simulink model "sim_main_esb_12"  (R2018b)
settings: Solver=VariableStepAuto  StartTime=0.0  StopTime=10  RelTol=1e-3
values from neighbouring files (symbols this model uses):
  A_klm = A_sys    [main_tf_12.m]    (also in main_tf_13.m = A_sys(1:6 , 1:6))
  B_klm = B_sys    [main_tf_12.m]    (also in main_tf_13.m = B_sys(1:6 , :))
  C = 0.344    [KALMAN.m]    (also in main_sys.m = double( subs( C) ); main_sys_klm.m = double( subs( C) ); main_tf_0.m = [ 0 , 0  , Ks , ds , -Ks , -ds, 0 ]; main_tf_1.m = C_mes)
  C_klm = C_sys    [main_tf_12.m]    (also in main_tf_13.m = C_sys(: , 1:6 ))
  Ct = double( subs( Ct) )    [main_sys.m]    (also in main_sys_klm.m; main_tf_10.m; main_tf_11.m; main_tf_12.m)
  D_klm = D_sys    [main_tf_12.m]    (also in main_tf_13.m)
  sys_sys = ss(A,B,C,D)    [main_sys.m]    (also in main_sys_klm.m; main_tf_10.m; main_tf_11.m; main_tf_12.m = ss(A_sys,B_sys,C_sys_mod,D_sys_mod))
undefined symbols (not defined in the file or in its folder): Continuous, K_lq, Time
libraries: ctrlSharedLib x1
settings Model: Creator=eshojaei  LastModifiedBy=eshojaei
settings CodeAppCC: StateflowObjectComments=on

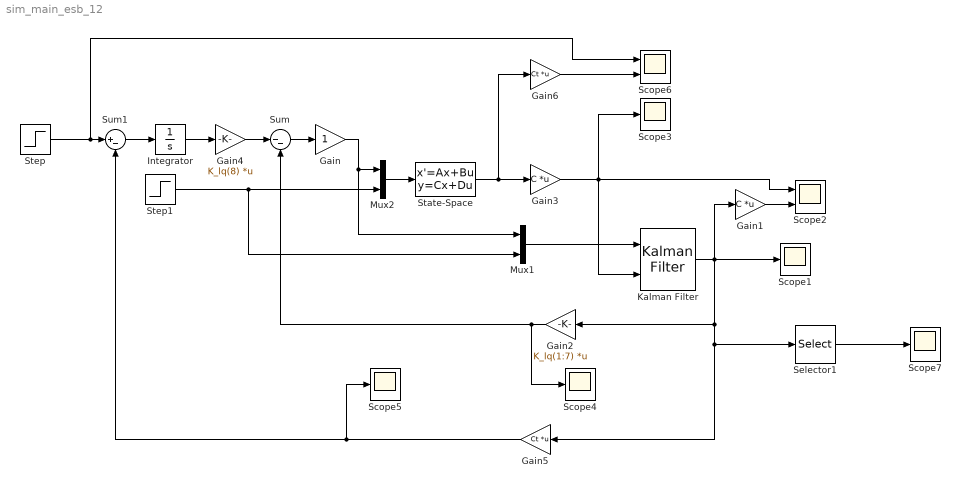
== system sim_main_esb_12 ==
  Gain : Gain
  Gain1 : Gain  Gain=C  Multiplication=Matrix(K*u)
  Gain2 : Gain  Gain=K_lq(1:7)  Multiplication=Matrix(K*u)
  Gain3 : Gain  Gain=C  Multiplication=Matrix(K*u)
  Gain4 : Gain  Gain=K_lq(8)  Multiplication=Matrix(K*u)
  Gain5 : Gain  Gain=Ct  Multiplication=Matrix(K*u)
  Gain6 : Gain  Gain=Ct  Multiplication=Matrix(K*u)
  Integrator : Integrator
  Kalman Filter : ctrlSharedLib/Kalman Filter  TimeDomain=Continuous-Time  UseCurrentEstimator=on  ModelSource=Individual A, B, C, D matrices  ModelSourceVariable=ss(0.95,1,1,0,1)  A=A_klm  B=B_klm  C=C_klm  D=D_klm  NumberOfStates=1  NumberOfInputs=1  NumberOfOutputs=1  InitialEstimateSource=Dialog  X0=0  P0=10  UseK=off  UseGH=off  NumberOfProcessNoiseInputs=1  G=1  TimeInvariantG=on  H=0  TimeInvariantH=on  Q=1  TimeInvariantQ=on  R=1  TimeInvariantR=on  N=0  TimeInvariantN=on  AddInputPort=on  AddEnablePort=off  OutputEstimatedY=off  OutputP=off  Ts=-1
      settings: SourceProductBaseCode=CT
  Mux1 : Mux  Inputs=2
  Mux2 : Mux  Inputs=2
  Scope{1,3..5,7} (5 alike) : Scope
  Scope2 : Scope  NumInputPorts=2
  Scope6 : Scope  NumInputPorts=2
  Selector1 : Selector  InputPortWidth=7  IndexOptions=Index vector (dialog)  Indices=[7]  OutputSizes=1
  State-Space : StateSpace  A=sys_sys.A  B=sys_sys.B  C=sys_sys.C  D=sys_sys.D  InitialCondition=0
  Step : Step  Time=.1  After=10  SampleTime=0
  Step1 : Step  Time=.1  After=.1  SampleTime=0
  Sum : Sum  Inputs=|--
  Sum1 : Sum  Inputs=|+-
  wires:
  Step1/1 -> Mux2/2, Mux1/2
  Gain3/1 -> Scope3/1, Scope2/1, Kalman Filter/2
  State-Space/1 -> Gain6/1, Gain3/1
  Mux1/1 -> Kalman Filter/1
  Mux2/1 -> State-Space/1
  Step/1 -> Scope6/1, Sum1/1
  Gain1/1 -> Scope2/2
  Gain2/1 -> Sum/2, Scope4/1
  Kalman Filter/1 -> Gain1/1, Gain2/1, Selector1/1, Gain5/1, Scope1/1
  Gain4/1 -> Sum/1
  Integrator/1 -> Gain4/1
  Sum1/1 -> Integrator/1
  Gain5/1 -> Scope5/1, Sum1/2
  Gain6/1 -> Scope6/2
  Sum/1 -> Gain/1
  Gain/1 -> Mux1/1, Mux2/1
  Selector1/1 -> Scope7/1
